simulink subsystem "QuadController"  (R2025a)
settings: Solver=VariableStepAuto  StartTime=0.0  StopTime=10.0  RelTol=1e-3
values from neighbouring files (symbols this model uses):
  b_0_pitch_ADRC = 463.821892393    [AttitudeControllers.mat]
  b_0_pitch_PDESO = 463.821892393    [AttitudeControllers.mat]
  b_0_roll_ADRC = 613.496932515    [AttitudeControllers.mat]
  b_0_roll_PDESO = 613.496932515    [AttitudeControllers.mat]
  b_0_x_ADRC = 1.53846153846    [PositionControllers.mat]
  b_0_x_PDESO = 1.53846153846    [PositionControllers.mat]
  b_0_y_ADRC = 1.53846153846    [PositionControllers.mat]
  b_0_y_PDESO = 1.53846153846    [PositionControllers.mat]
  b_0_yaw_ADRC = 304.785126486    [AttitudeControllers.mat]
  b_0_yaw_PDESO = 304.785126486    [AttitudeControllers.mat]
  b_0_z_ADRC = 1.53846153846    [PositionControllers.mat]
  b_0_z_PDESO = 1.53846153846    [PositionControllers.mat]
  L_ADRC_DT = [0.1032356623 -0.000431832114702 -0.000264667495719 0.74958434542 -0.00641793630067 -0.00397117455499 1.81400697556 -0.0234050723665 -0.0146188979088 -0.00057882817248 0.102990222012 0.000428820968351 ... (27 elements, 9x3)]    [AttitudeControllers.mat]
  L_ADRC_pos_DT = [0.0891378907785 -0.000524131917318 -0.0003553586831 0.554596680179 -0.00667403602859 -0.0045454658264 1.15001368908 -0.0209078013252 -0.0143041165707 -0.000577993893598 0.0890754257766 0.000256506390942 ... (27 elements, 9x3)]    [PositionControllers.mat]
  L_PDESO_DT = [0.1032356623 -0.000431832114702 -0.000264667495719 0.74958434542 -0.00641793630067 -0.00397117455499 1.81400697556 -0.0234050723665 -0.0146188979088 -0.00057882817248 0.102990222012 0.000428820968351 ... (27 elements, 9x3)]    [AttitudeControllers.mat]
  L_PDESO_pos_DT = [0.0459151556197 -7.78885413434e-05 0.000166988426468 0.143840448497 -0.000494397665849 0.00105523866626 0.150177599196 -0.000778075419383 0.00165361123935 -0.000147252211424 0.045775787359 -0.000280091532879 ... (27 elements, 9x3)]    [PositionControllers.mat]
  Ts_c = 0.005    [AttitudeControllers.mat]    (also in PositionControllers.mat)
  w_c_ADRC = 1.8    [AttitudeControllers.mat]
  w_c_ADRC_pos = 0.7    [PositionControllers.mat]
undefined symbols (not defined in the file or in its folder): A_eso, ADRC_ESO_DT, ADRC_ESO_pos_DT, b_0, b_0_x, b_0_y, b_0_z, B_eso, C_eso, d, ESO_CT, g, L_CT, m, PDESO_ESO_DT, PDESO_ESO_pos_DT, thrust2cmd, w_c, yaw2thrust
libraries: cstblocks x13, slctrl_disturbance x3, aerolibutil x3, matrix_library x1, dspmathops x1
settings Model: Creator=luker  LastModifiedBy=luke

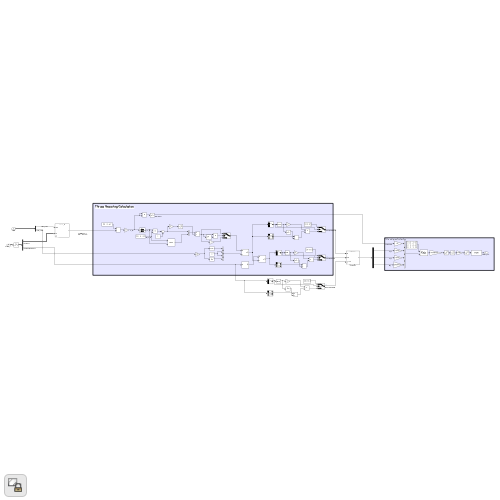
[thumbnail: Simulink's stored preview of the top-level diagram]
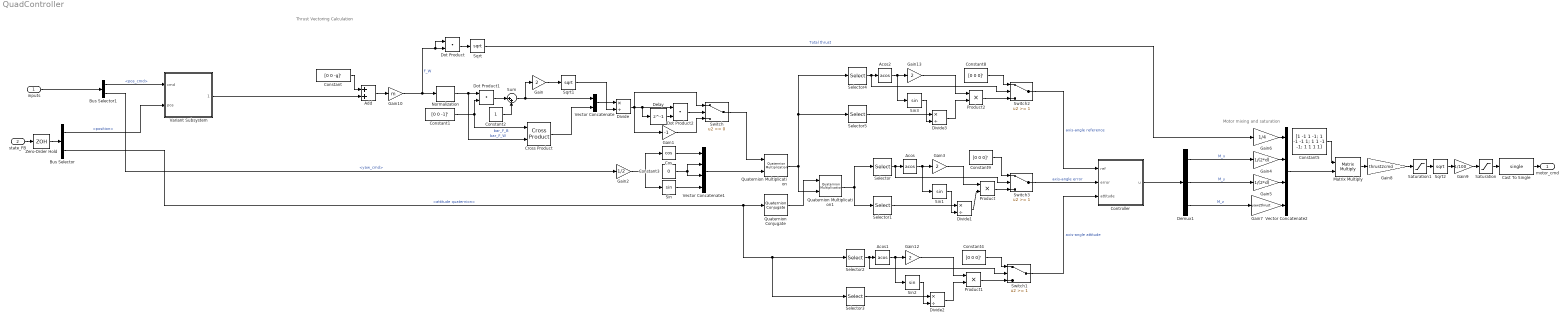
== system QuadController ==
  note: Motor mixing and saturation
  note: Thrust Vectoring Calculation
  inputs : Inport
  state_FB : Inport  Port=2
  Acos : Trigonometry  Operator=acos
  Acos1 : Trigonometry  Operator=acos
  Acos2 : Trigonometry  Operator=acos
  Add : Sum
  Bus Selector : BusSelector  OutputSignals=Translation State.position,Attitude State.attitude quaternion
  Bus Selector1 : BusSelector  OutputSignals=pos_cmd,yaw_cmd
  Cast To Single : DataTypeConversion  OutDataTypeStr=single  SaturateOnIntegerOverflow=off  RndMeth=Floor
  Constant : Constant  Value=[0 0 -g]'
  Constant1 : Constant  Value=[0 0 -1]'
  Constant2 : Constant
  Constant3 : Constant  Value=0
  Constant4 : Constant  Value=[0 0 0]'
  Constant5 : Constant  Value=[1 -1 1 -1; 1 -1 -1 1; 1 1 -1 -1; 1 1 1 1]
  Constant8 : Constant  Value=[0 0 0]'
  Constant9 : Constant  Value=[0 0 0]'
  Controller : Subsystem  Variant=on
  Cos : Trigonometry  Operator=cos
  Cross Product : matrix_library/Cross Product
  Delay : Delay  DelayLength=1
  Demux1 : Demux  Outputs=3
  Divide{,1..3} (4 alike) : Product  Inputs=*/
  Dot Product : DotProduct  OutDataTypeStr=Inherit: Inherit via internal rule
  Dot Product1 : DotProduct  OutDataTypeStr=Inherit: Inherit via internal rule
  Dot Product2 : DotProduct  OutDataTypeStr=Inherit: Inherit via internal rule
  Gain{,3,12..13} (4 alike) : Gain  Gain=2
  Gain1 : Gain  Gain=-1
  Gain10 : Gain  Gain=m
  Gain2 : Gain  Gain=1/2
  Gain4 : Gain  Gain=1/(2*d)
  Gain5 : Gain  Gain=1/(2*d)
  Gain6 : Gain  Gain=1/4
  Gain7 : Gain  Gain=yaw2thrust
  Gain8 : Gain  Gain=thrust2cmd
  Gain9 : Gain  Gain=1/100
  Matrix Multiply : Product  Multiplication=Matrix(*)
  Normalization : dspmathops/Normalization  NormType=2-norm  Bias=1e-10  NormOver=Each column  Dimension=1  roundingMode=Floor  overflowMode=off  accumDataTypeStr=Inherit: Same as product output  accumLastDataTypeStr=Inherit: Same as product output  outputDataTypeStr=Inherit: Same as product output  outputMin=[]  outputMax=[]  outputLastDataTypeStr=Inherit: Same as product output
  Product : Product
  Product1 : Product
  Product2 : Product
  Quaternion Conjugate : aerolibutil/Quaternion Conjugate
  Quaternion Multiplication : aerolibutil/Quaternion Multiplication
  Quaternion Multiplication1 : aerolibutil/Quaternion Multiplication
  Saturation : Saturate  UpperLimit=1  LowerLimit=0
  Saturation1 : Saturate  UpperLimit=inf  LowerLimit=0
  Selector : Selector  InputPortWidth=4  IndexOptions=Index vector (dialog)  Indices=1  OutputSizes=1
  Selector1 : Selector  InputPortWidth=4  IndexOptions=Index vector (dialog)  Indices=[2 3 4]  OutputSizes=1
  Selector2 : Selector  InputPortWidth=4  IndexOptions=Index vector (dialog)  Indices=1  OutputSizes=1
  Selector3 : Selector  InputPortWidth=4  IndexOptions=Index vector (dialog)  Indices=[2 3 4]  OutputSizes=1
  Selector4 : Selector  InputPortWidth=4  IndexOptions=Index vector (dialog)  Indices=1  OutputSizes=1
  Selector5 : Selector  InputPortWidth=4  IndexOptions=Index vector (dialog)  Indices=[2 3 4]  OutputSizes=1
  Sin{,1..3} (4 alike) : Trigonometry
  Sqrt : Sqrt
  Sqrt1 : Sqrt
  Sqrt2 : Sqrt
  Sum : Sum  Inputs=|++
  Switch : Switch  SaturateOnIntegerOverflow=off  InputSameDT=off
  Switch1 : Switch  Threshold=1  SaturateOnIntegerOverflow=off  InputSameDT=off
  Switch2 : Switch  Threshold=1  SaturateOnIntegerOverflow=off  InputSameDT=off
  Switch3 : Switch  Threshold=1  SaturateOnIntegerOverflow=off  InputSameDT=off
  Variant Subsystem : Subsystem  Variant=on
  Vector Concatenate : Concatenate
  Vector Concatenate1 : Concatenate  NumInputs=4
  Vector Concatenate2 : Concatenate  NumInputs=4
  Zero-Order Hold : ZeroOrderHold  SampleTime=Ts_c
  motor_cmd : Outport
  wires:
  Gain8/1 -> Saturation1/1
  state_FB/1 -> Zero-Order Hold/1
  Bus Selector1/2 -> Gain2/1  "<yaw_cmd>"
  Bus Selector/2 -> Quaternion Conjugate/1, Selector2/1, Selector3/1  "<attitude quaternion>"
  Constant/1 -> Add/1
  Add/1 -> Gain10/1
  Dot Product/1 -> Sqrt/1
  Sqrt/1 -> Gain6/1  "Total thrust"
  Constant1/1 -> Dot Product1/2, Cross Product/1  "bar_F_B"
  Normalization/1 -> Dot Product1/1, Cross Product/2  "bar_F_W"
  Dot Product1/1 -> Sum/1
  Constant2/1 -> Sum/2
  Sum/1 -> Gain/1, Vector Concatenate/1
  Gain/1 -> Sqrt1/1
  Cross Product/1 -> Vector Concatenate/2
  Vector Concatenate/1 -> Divide/1
  Sqrt1/1 -> Divide/2
  Dot Product2/1 -> Switch/2
  Divide/1 -> Switch/1, Gain1/1, Dot Product2/1, Delay/1
  Delay/1 -> Dot Product2/2
  Gain1/1 -> Switch/3
  Gain2/1 -> Sin/1, Cos/1
  Cos/1 -> Vector Concatenate1/1
  Sin/1 -> Vector Concatenate1/4
  Constant3/1 -> Vector Concatenate1/3, Vector Concatenate1/2
  Quaternion Conjugate/1 -> Quaternion Multiplication1/1
  Quaternion Multiplication/1 -> Selector4/1, Selector5/1, Quaternion Multiplication1/2
  Quaternion Multiplication1/1 -> Selector1/1, Selector/1
  Selector/1 -> Acos/1, Switch3/2
  Acos/1 -> Gain3/1, Sin1/1
  Selector1/1 -> Divide1/1
  Sin1/1 -> Divide1/2
  Gain3/1 -> Product/1
  Divide1/1 -> Product/2
  Gain6/1 -> Vector Concatenate2/1
  Gain4/1 -> Vector Concatenate2/2
  Gain5/1 -> Vector Concatenate2/3
  Gain7/1 -> Vector Concatenate2/4
  Constant5/1 -> Matrix Multiply/1
  Gain10/1 -> Normalization/1, Dot Product/2, Dot Product/1  "F_W"
  inputs/1 -> Bus Selector1/1
  Divide2/1 -> Product1/2
  Gain12/1 -> Product1/1
  Sin2/1 -> Divide2/2
  Selector3/1 -> Divide2/1
  Acos1/1 -> Sin2/1, Gain12/1
  Selector2/1 -> Acos1/1, Switch1/2
  Constant4/1 -> Switch1/1
  Switch1/1 -> Controller/3(attitude)  "axis-angle attitude"
  Product1/1 -> Switch1/3
  Divide3/1 -> Product2/2
  Sin3/1 -> Divide3/2
  Acos2/1 -> Sin3/1, Gain13/1
  Product2/1 -> Switch2/3
  Gain13/1 -> Product2/1
  Switch2/1 -> Controller/1(ref)  "axis-angle reference"
  Constant8/1 -> Switch2/1
  Selector4/1 -> Acos2/1, Switch2/2
  Selector5/1 -> Divide3/1
  Switch3/1 -> Controller/2(error)  "axis-angle error"
  Constant9/1 -> Switch3/1
  Product/1 -> Switch3/3
  Controller/1(u) -> Demux1/1
  Zero-Order Hold/1 -> Bus Selector/1
  Gain9/1 -> Saturation/1
  Sqrt2/1 -> Gain9/1
  Demux1/2 -> Gain5/1  "M_y"
  Vector Concatenate2/1 -> Matrix Multiply/2
  Saturation1/1 -> Sqrt2/1
  Matrix Multiply/1 -> Gain8/1
  Demux1/1 -> Gain4/1  "M_x"
  Demux1/3 -> Gain7/1  "M_z"
  Saturation/1 -> Cast To Single/1
  Cast To Single/1 -> motor_cmd/1
  Bus Selector1/1 -> Variant Subsystem/1(cmd)  "<pos_cmd>"
  Bus Selector/1 -> Variant Subsystem/2(pos)  "<position>"
  Variant Subsystem/1(1) -> Add/2
  Vector Concatenate1/1 -> Quaternion Multiplication/2
  Switch/1 -> Quaternion Multiplication/1

== system QuadController/Controller ==
  ref : Inport
  error : Inport  Port=2
  attitude : Inport  Port=3
  ADRC : Subsystem  VariantControl="AttController==\"1DOFADRC\""
  ADRC_3 : Subsystem  VariantControl="AttController==\"ADRC\""
  ADRC_3_CT : Subsystem  VariantControl="AttController==\"ADRC_CT\""
  Hinf : Subsystem  VariantControl="AttController==\"Hinf\""
  PD+ESO : Subsystem  VariantControl="AttController==\"PDESO\""
  PID : Subsystem  VariantControl="AttController==\"PID\""
  u : Outport

== system QuadController/Variant Subsystem ==
  cmd : Inport
  pos : Inport  Port=2
  ADRC_3 : Subsystem  VariantControl="PosController==\"ADRC\""
  AttitudeControl : Subsystem  VariantControl="PosController==\"none\""
  PD+ESO : Subsystem  VariantControl="PosController==\"PDESO\""
  PID : Subsystem  VariantControl="PosController==\"PID\""
  1 : Outport

== system QuadController/Controller/ADRC ==
  ref : Inport
  attitude : Inport  Port=2
  Demux : Demux  Outputs=3
  Demux1 : Demux  Outputs=3
  Mux : Mux  Inputs=3
  Subsystem1 : Subsystem
  Subsystem2 : Subsystem
  Subsystem3 : Subsystem
  u : Outport
  wires:
  Subsystem3/1(u) -> Mux/3
  Subsystem1/1(u) -> Mux/2
  Subsystem2/1(u) -> Mux/1
  Mux/1 -> u/1
  Demux1/3 -> Subsystem3/2(y)
  Demux/3 -> Subsystem3/1(r)
  Demux1/2 -> Subsystem1/2(y)
  Demux/2 -> Subsystem1/1(r)
  Demux1/1 -> Subsystem2/2(y)
  Demux/1 -> Subsystem2/1(r)
  attitude/1 -> Demux1/1
  ref/1 -> Demux/1

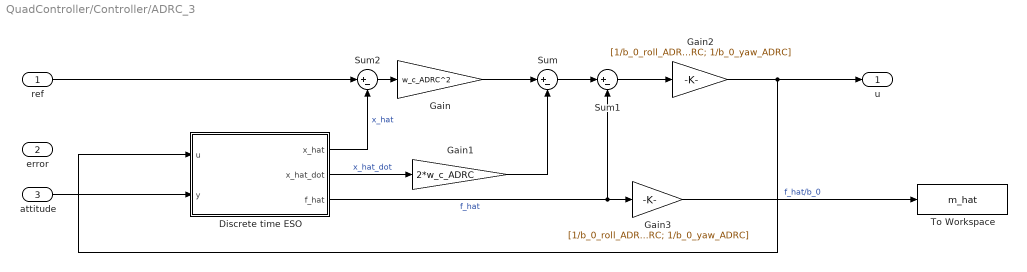
== system QuadController/Controller/ADRC_3 ==
  ref : Inport
  error : Inport  Port=2
  attitude : Inport  Port=3
  Discrete time ESO : Subsystem
  Gain : Gain  Gain=w_c_ADRC^2
  Gain1 : Gain  Gain=2*w_c_ADRC
  Gain2 : Gain  Gain=[1/b_0_roll_ADRC; 1/b_0_pitch_ADRC; 1/b_0_yaw_ADRC]
  Gain3 : Gain  Gain=[1/b_0_roll_ADRC; 1/b_0_pitch_ADRC; 1/b_0_yaw_ADRC]
  Sum : Sum  Inputs=|+-
  Sum1 : Sum  Inputs=|+-
  Sum2 : Sum  Inputs=|+-
  To Workspace : ToWorkspace  VariableName=m_hat  SaveFormat=Structure With Time  SampleTime=0.01
  u : Outport
  wires:
  Sum1/1 -> Gain2/1
  Sum/1 -> Sum1/1
  Gain1/1 -> Sum/2
  Discrete time ESO/2(x_hat_dot) -> Gain1/1  "x_hat_dot"
  Gain3/1 -> To Workspace/1  "f_hat/b_0"
  Gain2/1 -> u/1, Discrete time ESO/1(u)
  ref/1 -> Sum2/1
  Sum2/1 -> Gain/1
  attitude/1 -> Discrete time ESO/2(y)
  Discrete time ESO/3(f_hat) -> Sum1/2, Gain3/1  "f_hat"
  Gain/1 -> Sum/1
  Discrete time ESO/1(x_hat) -> Sum2/2  "x_hat"

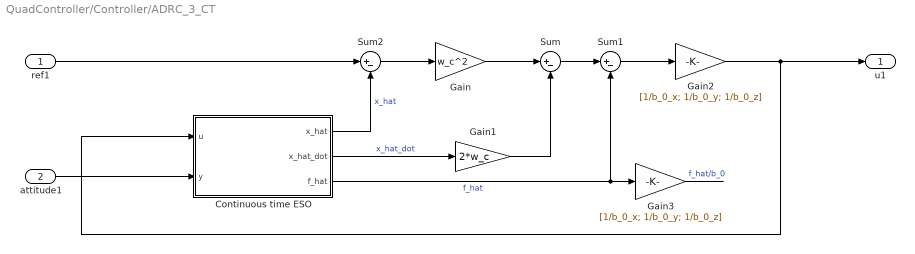
== system QuadController/Controller/ADRC_3_CT ==
  ref1 : Inport
  attitude1 : Inport  Port=2
  Continuous time ESO : Subsystem
  Gain : Gain  Gain=w_c^2
  Gain1 : Gain  Gain=2*w_c
  Gain2 : Gain  Gain=[1/b_0_x; 1/b_0_y; 1/b_0_z]
  Gain3 : Gain  Gain=[1/b_0_x; 1/b_0_y; 1/b_0_z]
  Sum : Sum  Inputs=|+-
  Sum1 : Sum  Inputs=|+-
  Sum2 : Sum  Inputs=|+-
  u1 : Outport
  wires:
  attitude1/1 -> Continuous time ESO/2(y)
  Continuous time ESO/3(f_hat) -> Sum1/2, Gain3/1  "f_hat"
  Sum1/1 -> Gain2/1
  Gain/1 -> Sum/1
  Continuous time ESO/1(x_hat) -> Sum2/2  "x_hat"
  Continuous time ESO/2(x_hat_dot) -> Gain1/1  "x_hat_dot"
  Gain1/1 -> Sum/2
  ref1/1 -> Sum2/1
  Gain3/1 -> ?  "f_hat/b_0"
  Sum2/1 -> Gain/1
  Sum/1 -> Sum1/1
  Gain2/1 -> u1/1, Continuous time ESO/1(u)

== system QuadController/Controller/Hinf ==
  error : Inport
  LTI System3 : cstblocks/LTI System  Commented=through  sys=G_hinf  IC=[]  PadeOrder=0
  u : Outport
  wires:
  error/1 -> LTI System3/1
  LTI System3/1 -> u/1

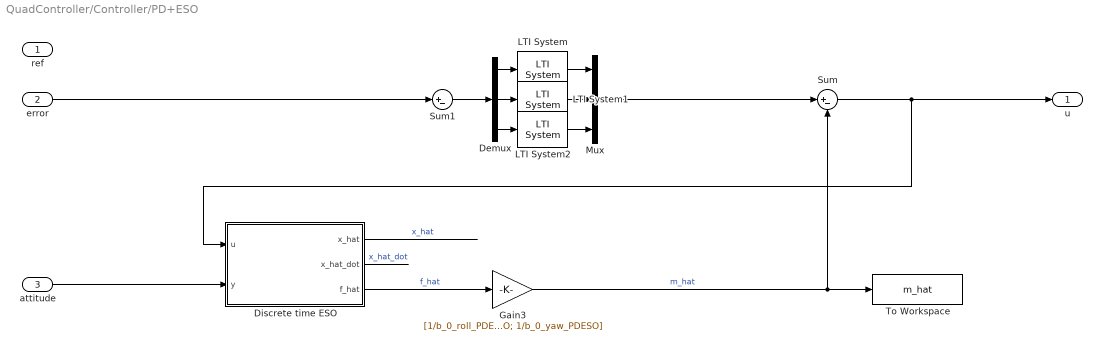
== system QuadController/Controller/PD+ESO ==
  ref : Inport
  error : Inport  Port=2
  attitude : Inport  Port=3
  Demux : Demux  Outputs=3
  Discrete time ESO : Subsystem
  Gain3 : Gain  Gain=[1/b_0_roll_PDESO; 1/b_0_pitch_PDESO; 1/b_0_yaw_PDESO]
  LTI System : cstblocks/LTI System  sys=G_PD_roll_DT  IC=[]  PadeOrder=0
  LTI System1 : cstblocks/LTI System  sys=G_PD_pitch_DT  IC=[]  PadeOrder=0
  LTI System2 : cstblocks/LTI System  sys=G_PD_yaw_DT  IC=[]  PadeOrder=0
  Mux : Mux  Inputs=3
  Sum : Sum  Inputs=|+-
  Sum1 : Sum  Inputs=|+-
  To Workspace : ToWorkspace  VariableName=m_hat  SaveFormat=Structure With Time  SampleTime=0.01
  u : Outport
  wires:
  Discrete time ESO/1(x_hat) -> ?  "x_hat"
  Discrete time ESO/2(x_hat_dot) -> ?  "x_hat_dot"
  error/1 -> Sum1/1
  Sum1/1 -> Demux/1
  Sum/1 -> u/1, Discrete time ESO/1(u)
  Mux/1 -> Sum/1
  LTI System2/1 -> Mux/3
  LTI System1/1 -> Mux/2
  LTI System/1 -> Mux/1
  Demux/2 -> LTI System1/1
  Demux/3 -> LTI System2/1
  Demux/1 -> LTI System/1
  Discrete time ESO/3(f_hat) -> Gain3/1  "f_hat"
  attitude/1 -> Discrete time ESO/2(y)
  Gain3/1 -> Sum/2, To Workspace/1  "m_hat"

== system QuadController/Controller/PID ==
  error : Inport
  Demux : Demux  Outputs=3
  LTI System : cstblocks/LTI System  sys=G_PID_roll_DT  IC=[]  PadeOrder=0
  LTI System1 : cstblocks/LTI System  sys=G_PID_pitch_DT  IC=[]  PadeOrder=0
  LTI System2 : cstblocks/LTI System  sys=G_PID_yaw_DT  IC=[]  PadeOrder=0
  Mux1 : Mux  Inputs=3
  u : Outport
  wires:
  error/1 -> Demux/1
  Demux/2 -> LTI System1/1
  Demux/1 -> LTI System/1
  LTI System/1 -> Mux1/1
  LTI System1/1 -> Mux1/2
  LTI System2/1 -> Mux1/3
  Mux1/1 -> u/1
  Demux/3 -> LTI System2/1

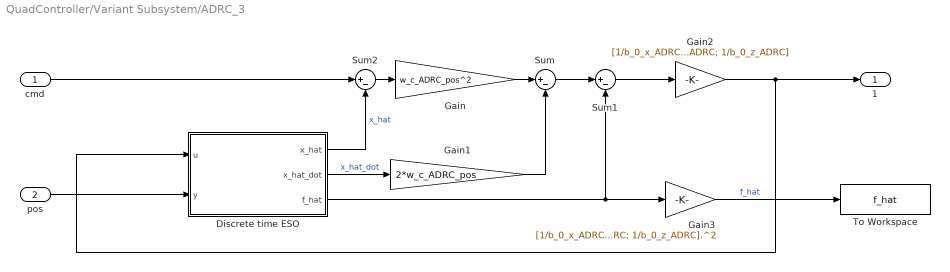
== system QuadController/Variant Subsystem/ADRC_3 ==
  cmd : Inport
  pos : Inport  Port=2
  Discrete time ESO : Subsystem
  Gain : Gain  Gain=w_c_ADRC_pos^2
  Gain1 : Gain  Gain=2*w_c_ADRC_pos
  Gain2 : Gain  Gain=[1/b_0_x_ADRC; 1/b_0_y_ADRC; 1/b_0_z_ADRC]
  Gain3 : Gain  Gain=[1/b_0_x_ADRC; 1/b_0_y_ADRC; 1/b_0_z_ADRC].^2
  Sum : Sum  Inputs=|+-
  Sum1 : Sum  Inputs=|+-
  Sum2 : Sum  Inputs=|+-
  To Workspace : ToWorkspace  VariableName=f_hat  SaveFormat=Structure With Time  SampleTime=0.01
  1 : Outport
  wires:
  Sum1/1 -> Gain2/1
  Sum/1 -> Sum1/1
  Gain1/1 -> Sum/2
  Discrete time ESO/2(x_hat_dot) -> Gain1/1  "x_hat_dot"
  Gain3/1 -> To Workspace/1  "f_hat"
  Gain2/1 -> 1/1, Discrete time ESO/1(u)
  cmd/1 -> Sum2/1
  Sum2/1 -> Gain/1
  pos/1 -> Discrete time ESO/2(y)
  Discrete time ESO/3(f_hat) -> Sum1/2, Gain3/1
  Gain/1 -> Sum/1
  Discrete time ESO/1(x_hat) -> Sum2/2  "x_hat"

== system QuadController/Variant Subsystem/AttitudeControl ==
  cmd : Inport
  pos : Inport  Port=2
  1 : Outport
  wires:
  cmd/1 -> 1/1

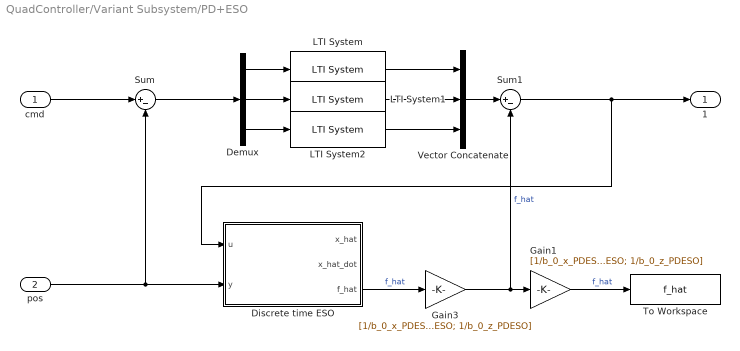
== system QuadController/Variant Subsystem/PD+ESO ==
  cmd : Inport
  pos : Inport  Port=2
  Demux : Demux  Outputs=3
  Discrete time ESO : Subsystem
  Gain1 : Gain  Gain=[1/b_0_x_PDESO; 1/b_0_y_PDESO; 1/b_0_z_PDESO]
  Gain3 : Gain  Gain=[1/b_0_x_PDESO; 1/b_0_y_PDESO; 1/b_0_z_PDESO]
  LTI System : cstblocks/LTI System  sys=G_PD_x_DT  IC=[]  PadeOrder=0
  LTI System1 : cstblocks/LTI System  sys=G_PD_y_DT  IC=[]  PadeOrder=0
  LTI System2 : cstblocks/LTI System  sys=G_PD_z_DT  IC=[]  PadeOrder=0
  Sum : Sum  Inputs=|+-
  Sum1 : Sum  Inputs=|+-
  To Workspace : ToWorkspace  VariableName=f_hat  SaveFormat=Structure With Time  SampleTime=0.01
  Vector Concatenate : Concatenate  NumInputs=3
  1 : Outport
  wires:
  Gain1/1 -> To Workspace/1  "f_hat"
  Gain3/1 -> Sum1/2, Gain1/1  "f_hat"
  Discrete time ESO/3(f_hat) -> Gain3/1  "f_hat"
  Sum1/1 -> 1/1, Discrete time ESO/1(u)
  Vector Concatenate/1 -> Sum1/1
  pos/1 -> Sum/2, Discrete time ESO/2(y)
  cmd/1 -> Sum/1
  Sum/1 -> Demux/1
  LTI System/1 -> Vector Concatenate/1
  Demux/2 -> LTI System1/1
  Demux/1 -> LTI System/1
  Demux/3 -> LTI System2/1
  LTI System2/1 -> Vector Concatenate/3
  LTI System1/1 -> Vector Concatenate/2

== system QuadController/Variant Subsystem/PID ==
  cmd : Inport
  pos : Inport  Port=2
  Demux : Demux  Outputs=3
  LTI System : cstblocks/LTI System  sys=G_PID_x_DT  IC=[]  PadeOrder=0
  LTI System1 : cstblocks/LTI System  sys=G_PID_y_DT  IC=[]  PadeOrder=0
  LTI System2 : cstblocks/LTI System  sys=G_PID_z_DT  IC=[]  PadeOrder=0
  Sum : Sum  Inputs=|+-
  Vector Concatenate : Concatenate  NumInputs=3
  1 : Outport
  wires:
  pos/1 -> Sum/2
  cmd/1 -> Sum/1
  Sum/1 -> Demux/1
  LTI System/1 -> Vector Concatenate/1
  LTI System1/1 -> Vector Concatenate/2
  Vector Concatenate/1 -> 1/1
  Demux/3 -> LTI System2/1
  Demux/1 -> LTI System/1
  LTI System2/1 -> Vector Concatenate/3
  Demux/2 -> LTI System1/1

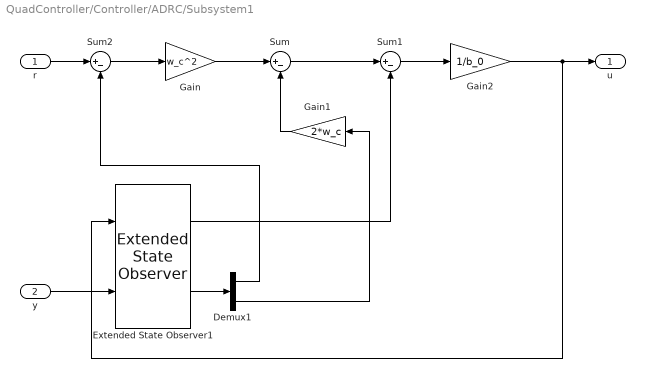
== system QuadController/Controller/ADRC/Subsystem1 ==
  r : Inport
  y : Inport  Port=2
  Demux1 : Demux  Outputs=2
  Extended State Observer1 : slctrl_disturbance/Extended State Observer  time_domain=continuous-time  Ts=1/250  sys=ss(A_eso,B_eso,C_eso,zeros(1,1))  model_ext=off  nx=2  nu=1  ny=1  k=1/b_0  Bd_ext=off  nd=1  s0=0  s0_ext=off  wo=w_o  delta=0.01  L_ext=off  data_type=double  hasDelay=off  Td=1  output_xhat=on
      settings: LibrarySourceBlock=slctrlblks/Disturbance Observer/Extended State Observer
  Gain : Gain  Gain=w_c^2
  Gain1 : Gain  Gain=2*w_c
  Gain2 : Gain  Gain=1/b_0
  Sum : Sum  Inputs=|+-
  Sum1 : Sum  Inputs=|+-
  Sum2 : Sum  Inputs=|+-
  u : Outport
  wires:
  Extended State Observer1/2 -> Demux1/1
  Gain/1 -> Sum/1
  Gain1/1 -> Sum/2
  Gain2/1 -> u/1, Extended State Observer1/1
  Sum/1 -> Sum1/1
  Sum1/1 -> Gain2/1
  Extended State Observer1/1 -> Sum1/2
  Demux1/2 -> Gain1/1
  y/1 -> Extended State Observer1/2
  r/1 -> Sum2/1
  Sum2/1 -> Gain/1
  Demux1/1 -> Sum2/2

== system QuadController/Controller/ADRC/Subsystem2 ==
  r : Inport
  y : Inport  Port=2
  Demux1 : Demux  Outputs=2
  Extended State Observer1 : slctrl_disturbance/Extended State Observer  time_domain=continuous-time  Ts=1/250  sys=ss(A_eso,B_eso,C_eso,zeros(1,1))  model_ext=off  nx=2  nu=1  ny=1  k=1/b_0  Bd_ext=off  nd=1  s0=0  s0_ext=off  wo=w_o  delta=0.01  L_ext=off  data_type=double  hasDelay=off  Td=1  output_xhat=on
      settings: LibrarySourceBlock=slctrlblks/Disturbance Observer/Extended State Observer
  Gain : Gain  Gain=w_c^2
  Gain1 : Gain  Gain=2*w_c
  Gain2 : Gain  Gain=1/b_0
  Sum : Sum  Inputs=|+-
  Sum1 : Sum  Inputs=|+-
  Sum2 : Sum  Inputs=|+-
  u : Outport
  wires:
  Demux1/1 -> Sum2/2
  Sum2/1 -> Gain/1
  r/1 -> Sum2/1
  y/1 -> Extended State Observer1/2
  Demux1/2 -> Gain1/1
  Extended State Observer1/1 -> Sum1/2
  Sum1/1 -> Gain2/1
  Sum/1 -> Sum1/1
  Gain2/1 -> Extended State Observer1/1, u/1
  Gain1/1 -> Sum/2
  Gain/1 -> Sum/1
  Extended State Observer1/2 -> Demux1/1

== system QuadController/Controller/ADRC/Subsystem3 ==
  r : Inport
  y : Inport  Port=2
  Demux1 : Demux  Outputs=2
  Extended State Observer1 : slctrl_disturbance/Extended State Observer  time_domain=continuous-time  Ts=1/250  sys=ss(A_eso,B_eso,C_eso,zeros(1,1))  model_ext=off  nx=2  nu=1  ny=1  k=1/b_0  Bd_ext=off  nd=1  s0=0  s0_ext=off  wo=w_o  delta=0.01  L_ext=off  data_type=double  hasDelay=off  Td=1  output_xhat=on
      settings: LibrarySourceBlock=slctrlblks/Disturbance Observer/Extended State Observer
  Gain : Gain  Gain=w_c^2
  Gain1 : Gain  Gain=2*w_c
  Gain2 : Gain  Gain=1/b_0
  Sum : Sum  Inputs=|+-
  Sum1 : Sum  Inputs=|+-
  Sum2 : Sum  Inputs=|+-
  u : Outport
  wires:
  Demux1/1 -> Sum2/2
  Sum2/1 -> Gain/1
  r/1 -> Sum2/1
  y/1 -> Extended State Observer1/2
  Demux1/2 -> Gain1/1
  Extended State Observer1/1 -> Sum1/2
  Sum1/1 -> Gain2/1
  Sum/1 -> Sum1/1
  Gain2/1 -> Extended State Observer1/1, u/1
  Gain1/1 -> Sum/2
  Gain/1 -> Sum/1
  Extended State Observer1/2 -> Demux1/1

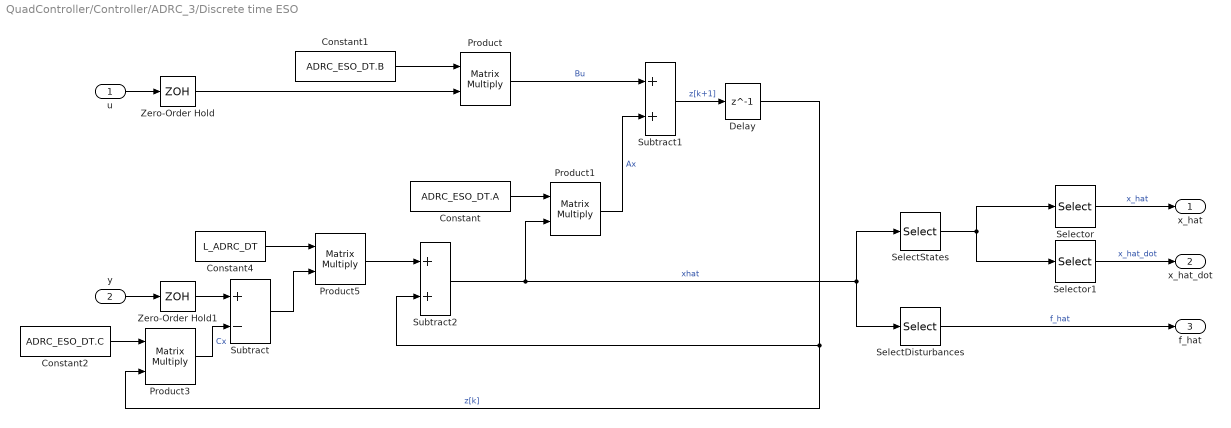
== system QuadController/Controller/ADRC_3/Discrete time ESO ==
  u : Inport
  y : Inport  Port=2
  Constant : Constant  Value=ADRC_ESO_DT.A
  Constant1 : Constant  Value=ADRC_ESO_DT.B
  Constant2 : Constant  Value=ADRC_ESO_DT.C
  Constant4 : Constant  Value=L_ADRC_DT
  Delay : Delay  DelayLength=1  InitialCondition=[0 0 0 0 0 0 0 0 0]'  SampleTime=Ts_c
  Product{,1,3,5} (4 alike) : Product  SCDEnableBlockLinearizationSpecification=on  Multiplication=Matrix(*)
  SelectDisturbances : Selector  InputPortWidth=9  IndexOptions=Index vector (dialog)  Indices=6+1:6+3  OutputSizes=1
  SelectStates : Selector  InputPortWidth=9  IndexOptions=Index vector (dialog)  Indices=[1:6]  OutputSizes=1
  Selector : Selector  InputPortWidth=6  IndexOptions=Index vector (dialog)  Indices=[1 2 3]  OutputSizes=1
  Selector1 : Selector  InputPortWidth=6  IndexOptions=Index vector (dialog)  Indices=[4 5 6]  OutputSizes=1
  Subtract : Sum  Inputs=+-
  Subtract1 : Sum
  Subtract2 : Sum
  Zero-Order Hold : ZeroOrderHold  SampleTime=Ts_c
  Zero-Order Hold1 : ZeroOrderHold  SampleTime=Ts_c
  x_hat : Outport
  x_hat_dot : Outport  Port=2
  f_hat : Outport  Port=3
  wires:
  Zero-Order Hold1/1 -> Subtract/1
  Zero-Order Hold/1 -> Product/2
  Selector1/1 -> x_hat_dot/1  "x_hat_dot"
  Selector/1 -> x_hat/1  "x_hat"
  SelectDisturbances/1 -> f_hat/1  "f_hat"
  SelectStates/1 -> Selector/1, Selector1/1
  Product/1 -> Subtract1/1  "Bu"
  Subtract/1 -> Product5/2
  Product3/1 -> Subtract/2  "Cx"
  Product5/1 -> Subtract2/1
  Constant2/1 -> Product3/1
  u/1 -> Zero-Order Hold/1
  Subtract2/1 -> SelectDisturbances/1, SelectStates/1, Product1/2  "xhat"
  Constant/1 -> Product1/1
  Constant1/1 -> Product/1
  Constant4/1 -> Product5/1
  Product1/1 -> Subtract1/2  "Ax"
  Delay/1 -> Product3/2, Subtract2/2  "z[k]"
  Subtract1/1 -> Delay/1  "z[k+1]"
  y/1 -> Zero-Order Hold1/1

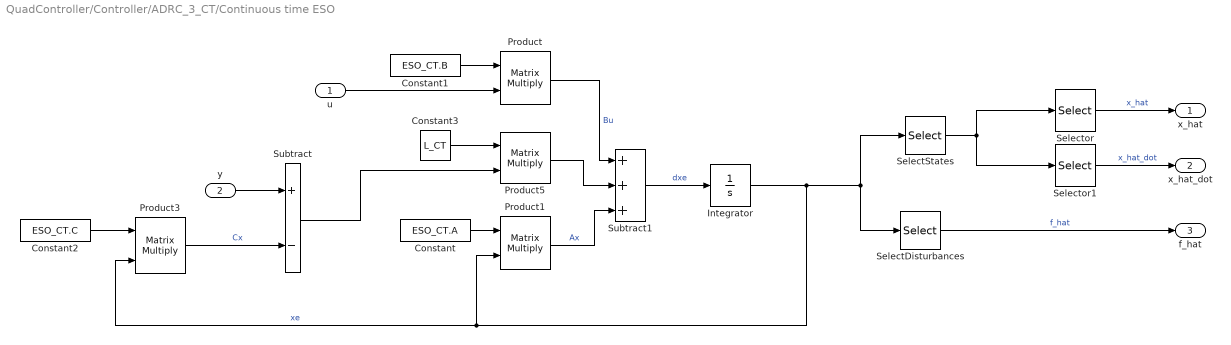
== system QuadController/Controller/ADRC_3_CT/Continuous time ESO ==
  u : Inport
  y : Inport  Port=2
  Constant : Constant  Value=ESO_CT.A
  Constant1 : Constant  Value=ESO_CT.B
  Constant2 : Constant  Value=ESO_CT.C
  Constant3 : Constant  Value=L_CT
  Integrator : Integrator  InitialCondition=[0 0 0 0 0 0 0 0 0]
  Product{,1,3,5} (4 alike) : Product  SCDEnableBlockLinearizationSpecification=on  Multiplication=Matrix(*)
  SelectDisturbances : Selector  InputPortWidth=9  IndexOptions=Index vector (dialog)  Indices=6+1:6+3  OutputSizes=1
  SelectStates : Selector  InputPortWidth=9  IndexOptions=Index vector (dialog)  Indices=[1:6]  OutputSizes=1
  Selector : Selector  InputPortWidth=6  IndexOptions=Index vector (dialog)  Indices=[1 2 3]  OutputSizes=1
  Selector1 : Selector  InputPortWidth=6  IndexOptions=Index vector (dialog)  Indices=[4 5 6]  OutputSizes=1
  Subtract : Sum  Inputs=+-
  Subtract1 : Sum  Inputs=+++
  x_hat : Outport
  x_hat_dot : Outport  Port=2
  f_hat : Outport  Port=3
  wires:
  Selector/1 -> x_hat/1  "x_hat"
  SelectDisturbances/1 -> f_hat/1  "f_hat"
  SelectStates/1 -> Selector/1, Selector1/1
  Selector1/1 -> x_hat_dot/1  "x_hat_dot"
  Product/1 -> Subtract1/1  "Bu"
  Product5/1 -> Subtract1/2
  Subtract1/1 -> Integrator/1  "dxe"
  Constant2/1 -> Product3/1
  y/1 -> Subtract/1
  Integrator/1 -> Product3/2, Product1/2, SelectDisturbances/1, SelectStates/1  "xe"
  Constant3/1 -> Product5/1
  Constant1/1 -> Product/1
  Subtract/1 -> Product5/2
  Product3/1 -> Subtract/2  "Cx"
  u/1 -> Product/2
  Constant/1 -> Product1/1
  Product1/1 -> Subtract1/3  "Ax"

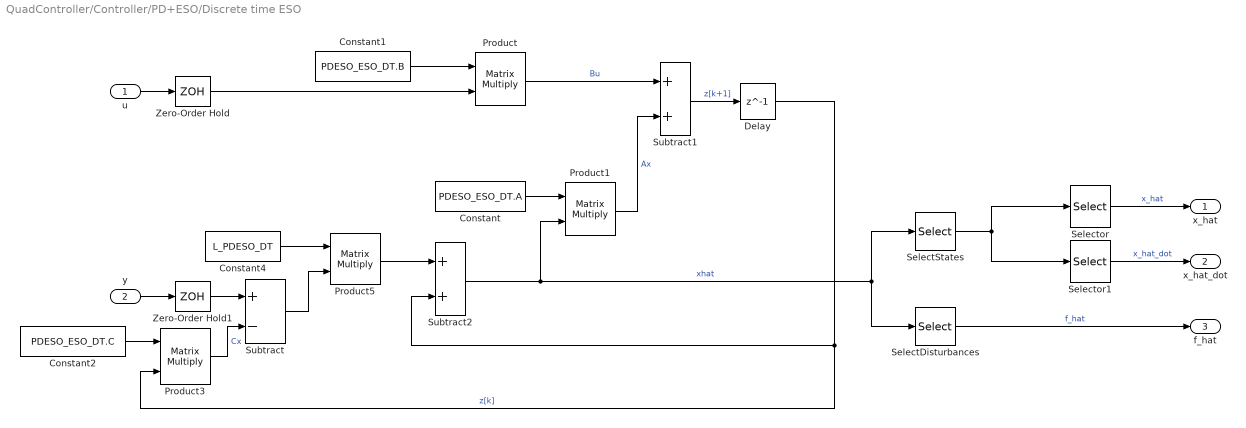
== system QuadController/Controller/PD+ESO/Discrete time ESO ==
  u : Inport
  y : Inport  Port=2
  Constant : Constant  Value=PDESO_ESO_DT.A
  Constant1 : Constant  Value=PDESO_ESO_DT.B
  Constant2 : Constant  Value=PDESO_ESO_DT.C
  Constant4 : Constant  Value=L_PDESO_DT
  Delay : Delay  DelayLength=1  InitialCondition=[0 0 0 0 0 0 0 0 0]'  SampleTime=Ts_c
  Product{,1,3,5} (4 alike) : Product  SCDEnableBlockLinearizationSpecification=on  Multiplication=Matrix(*)
  SelectDisturbances : Selector  InputPortWidth=9  IndexOptions=Index vector (dialog)  Indices=6+1:6+3  OutputSizes=1
  SelectStates : Selector  InputPortWidth=9  IndexOptions=Index vector (dialog)  Indices=[1:6]  OutputSizes=1
  Selector : Selector  InputPortWidth=6  IndexOptions=Index vector (dialog)  Indices=[1 2 3]  OutputSizes=1
  Selector1 : Selector  InputPortWidth=6  IndexOptions=Index vector (dialog)  Indices=[4 5 6]  OutputSizes=1
  Subtract : Sum  Inputs=+-
  Subtract1 : Sum
  Subtract2 : Sum
  Zero-Order Hold : ZeroOrderHold  SampleTime=Ts_c
  Zero-Order Hold1 : ZeroOrderHold  SampleTime=Ts_c
  x_hat : Outport
  x_hat_dot : Outport  Port=2
  f_hat : Outport  Port=3
  wires:
  Zero-Order Hold1/1 -> Subtract/1
  Zero-Order Hold/1 -> Product/2
  Selector1/1 -> x_hat_dot/1  "x_hat_dot"
  Selector/1 -> x_hat/1  "x_hat"
  SelectDisturbances/1 -> f_hat/1  "f_hat"
  SelectStates/1 -> Selector/1, Selector1/1
  Product/1 -> Subtract1/1  "Bu"
  Subtract/1 -> Product5/2
  Product3/1 -> Subtract/2  "Cx"
  Product5/1 -> Subtract2/1
  Constant2/1 -> Product3/1
  u/1 -> Zero-Order Hold/1
  Subtract2/1 -> SelectDisturbances/1, SelectStates/1, Product1/2  "xhat"
  Constant/1 -> Product1/1
  Constant1/1 -> Product/1
  Constant4/1 -> Product5/1
  Product1/1 -> Subtract1/2  "Ax"
  Delay/1 -> Product3/2, Subtract2/2  "z[k]"
  Subtract1/1 -> Delay/1  "z[k+1]"
  y/1 -> Zero-Order Hold1/1

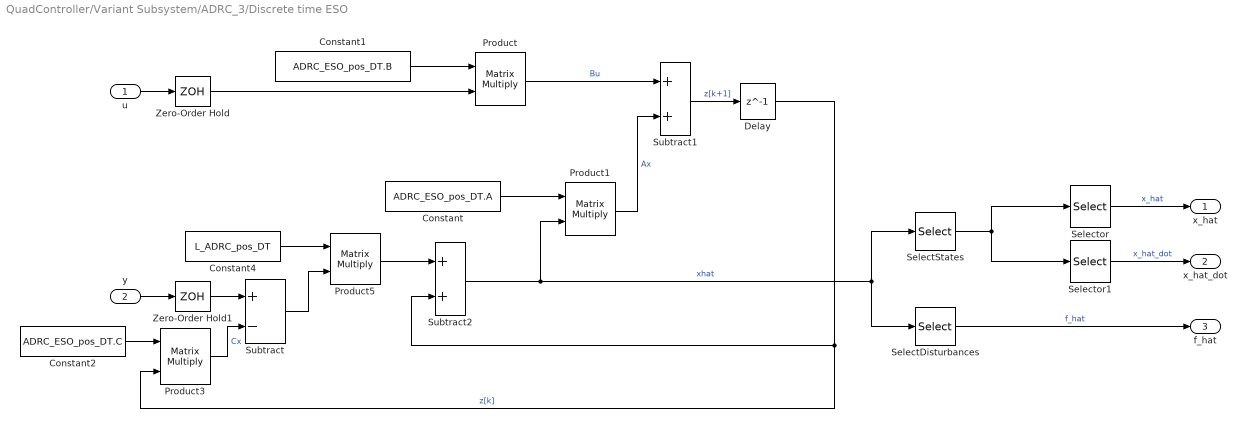
== system QuadController/Variant Subsystem/ADRC_3/Discrete time ESO ==
  u : Inport
  y : Inport  Port=2
  Constant : Constant  Value=ADRC_ESO_pos_DT.A
  Constant1 : Constant  Value=ADRC_ESO_pos_DT.B
  Constant2 : Constant  Value=ADRC_ESO_pos_DT.C
  Constant4 : Constant  Value=L_ADRC_pos_DT
  Delay : Delay  DelayLength=1  InitialCondition=[0 0 0 0 0 0 0 0 0]'  SampleTime=Ts_c
  Product{,1,3,5} (4 alike) : Product  SCDEnableBlockLinearizationSpecification=on  Multiplication=Matrix(*)
  SelectDisturbances : Selector  InputPortWidth=9  IndexOptions=Index vector (dialog)  Indices=6+1:6+3  OutputSizes=1
  SelectStates : Selector  InputPortWidth=9  IndexOptions=Index vector (dialog)  Indices=[1:6]  OutputSizes=1
  Selector : Selector  InputPortWidth=6  IndexOptions=Index vector (dialog)  Indices=[1 2 3]  OutputSizes=1
  Selector1 : Selector  InputPortWidth=6  IndexOptions=Index vector (dialog)  Indices=[4 5 6]  OutputSizes=1
  Subtract : Sum  Inputs=+-
  Subtract1 : Sum
  Subtract2 : Sum
  Zero-Order Hold : ZeroOrderHold  SampleTime=Ts_c
  Zero-Order Hold1 : ZeroOrderHold  SampleTime=Ts_c
  x_hat : Outport
  x_hat_dot : Outport  Port=2
  f_hat : Outport  Port=3
  wires:
  Zero-Order Hold1/1 -> Subtract/1
  Zero-Order Hold/1 -> Product/2
  Selector1/1 -> x_hat_dot/1  "x_hat_dot"
  Selector/1 -> x_hat/1  "x_hat"
  SelectDisturbances/1 -> f_hat/1  "f_hat"
  SelectStates/1 -> Selector/1, Selector1/1
  Product/1 -> Subtract1/1  "Bu"
  Subtract/1 -> Product5/2
  Product3/1 -> Subtract/2  "Cx"
  Product5/1 -> Subtract2/1
  Constant2/1 -> Product3/1
  u/1 -> Zero-Order Hold/1
  Subtract2/1 -> SelectDisturbances/1, SelectStates/1, Product1/2  "xhat"
  Constant/1 -> Product1/1
  Constant1/1 -> Product/1
  Constant4/1 -> Product5/1
  Product1/1 -> Subtract1/2  "Ax"
  Delay/1 -> Product3/2, Subtract2/2  "z[k]"
  Subtract1/1 -> Delay/1  "z[k+1]"
  y/1 -> Zero-Order Hold1/1

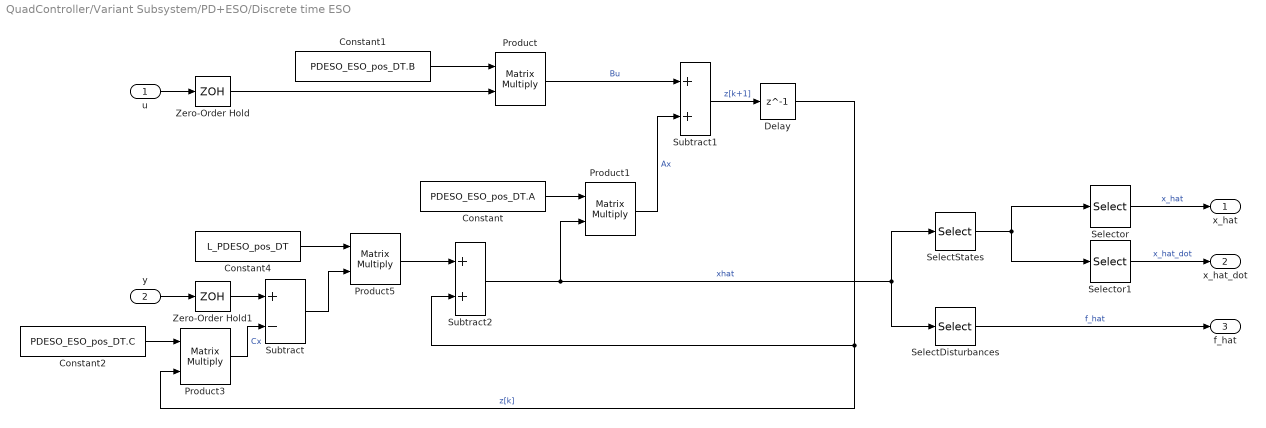
== system QuadController/Variant Subsystem/PD+ESO/Discrete time ESO ==
  u : Inport
  y : Inport  Port=2
  Constant : Constant  Value=PDESO_ESO_pos_DT.A
  Constant1 : Constant  Value=PDESO_ESO_pos_DT.B
  Constant2 : Constant  Value=PDESO_ESO_pos_DT.C
  Constant4 : Constant  Value=L_PDESO_pos_DT
  Delay : Delay  DelayLength=1  InitialCondition=[0 0 0 0 0 0 0 0 0]'  SampleTime=Ts_c
  Product{,1,3,5} (4 alike) : Product  SCDEnableBlockLinearizationSpecification=on  Multiplication=Matrix(*)
  SelectDisturbances : Selector  InputPortWidth=9  IndexOptions=Index vector (dialog)  Indices=6+1:6+3  OutputSizes=1
  SelectStates : Selector  InputPortWidth=9  IndexOptions=Index vector (dialog)  Indices=[1:6]  OutputSizes=1
  Selector : Selector  InputPortWidth=6  IndexOptions=Index vector (dialog)  Indices=[1 2 3]  OutputSizes=1
  Selector1 : Selector  InputPortWidth=6  IndexOptions=Index vector (dialog)  Indices=[4 5 6]  OutputSizes=1
  Subtract : Sum  Inputs=+-
  Subtract1 : Sum
  Subtract2 : Sum
  Zero-Order Hold : ZeroOrderHold  SampleTime=Ts_c
  Zero-Order Hold1 : ZeroOrderHold  SampleTime=Ts_c
  x_hat : Outport
  x_hat_dot : Outport  Port=2
  f_hat : Outport  Port=3
  wires:
  Zero-Order Hold1/1 -> Subtract/1
  Zero-Order Hold/1 -> Product/2
  Selector1/1 -> x_hat_dot/1  "x_hat_dot"
  Selector/1 -> x_hat/1  "x_hat"
  SelectDisturbances/1 -> f_hat/1  "f_hat"
  SelectStates/1 -> Selector/1, Selector1/1
  Product/1 -> Subtract1/1  "Bu"
  Subtract/1 -> Product5/2
  Product3/1 -> Subtract/2  "Cx"
  Product5/1 -> Subtract2/1
  Constant2/1 -> Product3/1
  u/1 -> Zero-Order Hold/1
  Subtract2/1 -> SelectDisturbances/1, SelectStates/1, Product1/2  "xhat"
  Constant/1 -> Product1/1
  Constant1/1 -> Product/1
  Constant4/1 -> Product5/1
  Product1/1 -> Subtract1/2  "Ax"
  Delay/1 -> Product3/2, Subtract2/2  "z[k]"
  Subtract1/1 -> Delay/1  "z[k+1]"
  y/1 -> Zero-Order Hold1/1
